simulink subsystem "sin_abs"  (R2022b)
settings: Solver=VariableStepAuto  StartTime=0.0  StopTime=10.0  RelTol=1e-3
settings Model: Creator=User  LastModifiedBy=User

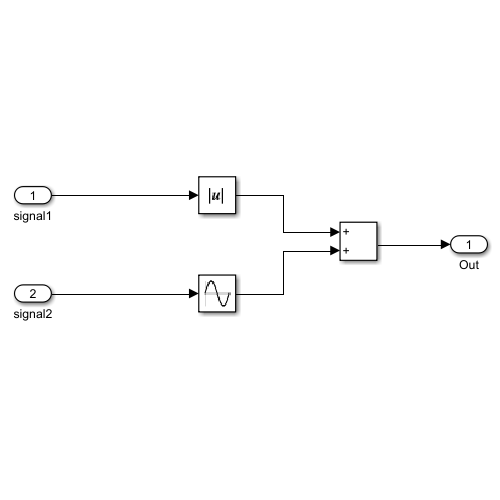
[thumbnail: Simulink's stored preview of the top-level diagram]
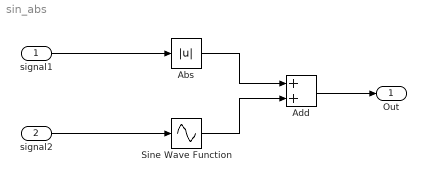
== system sin_abs ==
  signal1 : Inport
  signal2 : Inport  Port=2
  Abs : Abs  SaturateOnIntegerOverflow=off
  Add : Sum
  Sine Wave Function : Sin  TimeSource=Use external signal  SampleTime=0
  Out : Outport
  wires:
  signal1/1 -> Abs/1
  signal2/1 -> Sine Wave Function/1
  Sine Wave Function/1 -> Add/2
  Abs/1 -> Add/1
  Add/1 -> Out/1
